simulink model "ame532Project1_onedrive"  (R2022a)
settings: Solver=ode4  StartTime=0.0  StopTime=120  FixedStep=0.01  RelTol=1e-3
model workspace (MAT data in the model file):
  theta = Simulink.Parameter
  theta.DataType = 'auto'
  theta.Complexity = 'real'
  theta.Dimensions = [0 0]
undefined symbols (not defined in the file): earthRadius
libraries: simulink_extras x11, matrix_library x6, aerolibfltsims x2, vrlib x1, aerolibtransform2 x1, aerolibutil x1
(part 1 of 2)
settings Model: Creator=enson  LastModifiedBy=enson

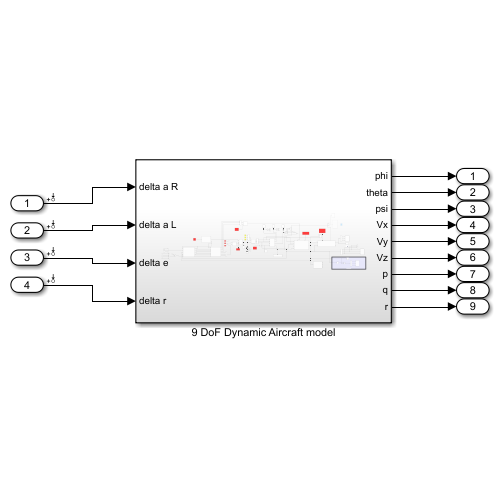
[thumbnail: Simulink's stored preview of the top-level diagram]
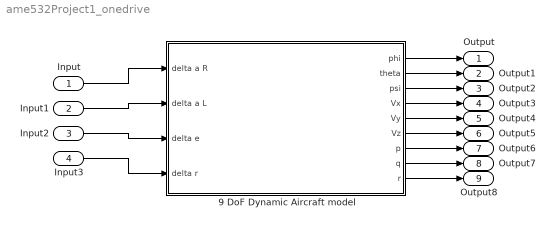
== system ame532Project1_onedrive ==
  Input : Inport
  Input1 : Inport  Port=2
  Input2 : Inport  Port=3
  Input3 : Inport  Port=4
  9 DoF Dynamic Aircraft model : Subsystem
  Output : Outport
  Output1 : Outport  Port=2
  Output2 : Outport  Port=3
  Output3 : Outport  Port=4
  Output4 : Outport  Port=5
  Output5 : Outport  Port=6
  Output6 : Outport  Port=7
  Output7 : Outport  Port=8
  Output8 : Outport  Port=9
  wires:
  Input/1 -> 9 DoF Dynamic Aircraft model/1(delta a R)
  Input1/1 -> 9 DoF Dynamic Aircraft model/2(delta a L)
  Input2/1 -> 9 DoF Dynamic Aircraft model/3(delta e)
  Input3/1 -> 9 DoF Dynamic Aircraft model/4(delta r)
  9 DoF Dynamic Aircraft model/1(phi) -> Output/1
  9 DoF Dynamic Aircraft model/2(theta) -> Output1/1
  9 DoF Dynamic Aircraft model/3(psi) -> Output2/1
  9 DoF Dynamic Aircraft model/4(Vx) -> Output3/1
  9 DoF Dynamic Aircraft model/5(Vy) -> Output4/1
  9 DoF Dynamic Aircraft model/6(Vz) -> Output5/1
  9 DoF Dynamic Aircraft model/7(p) -> Output6/1
  9 DoF Dynamic Aircraft model/8(q) -> Output7/1
  9 DoF Dynamic Aircraft model/9(r) -> Output8/1

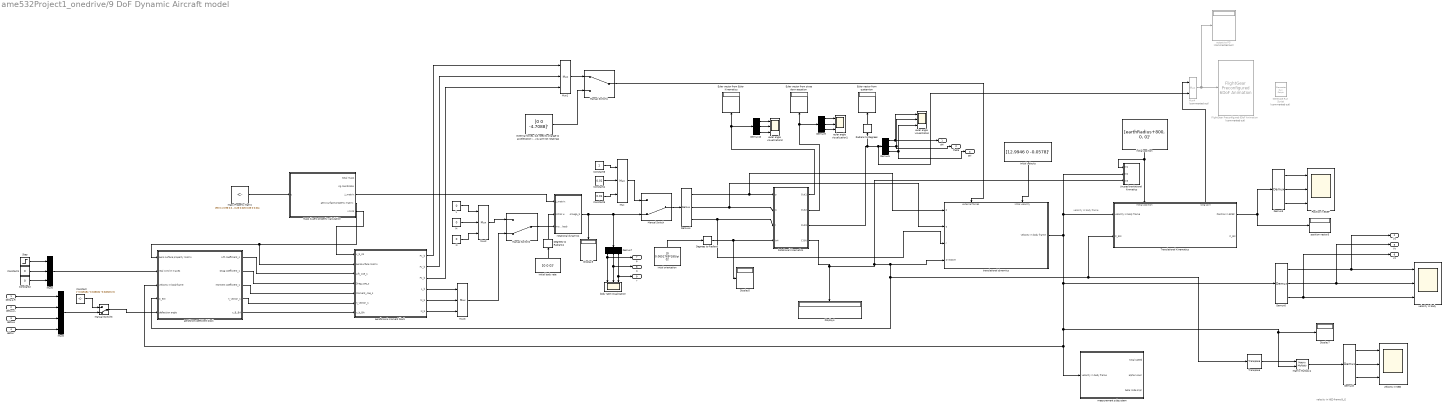
== system ame532Project1_onedrive/9 DoF Dynamic Aircraft model ==
  note: velocity in NED frame B_E
  note: velocity in body frame
  delta a R : Inport
  delta a L : Inport  Port=2
  delta e : Inport  Port=3
  delta r : Inport  Port=4
  Constant : Constant  Value=[-0.046184 -0.046184 -0.048101 0]
  Constant1 : Constant  Value=0
  Constant2 : Constant  Value=0
  Constant4 : Constant  Value=0.01
  Constant5 : Constant  Value=0.01
  Constant6 : Constant
  Degrees to Radians : simulink_extras/Transformations/Degrees to Radians
  Degrees to Radians1 : simulink_extras/Transformations/Degrees to Radians
  Demux{3..10} (8 alike) : Demux  Outputs=3
  Display{3..5,7} (4 alike) : Display
  Euler vector from Euler Kinematics : Display
  Euler vector from quaternion : Display
  Euler vector from strap down equation : Display
  FlightGear Preconfigured 6DoF Animation : aerolibfltsims/FlightGear Preconfigured 6DoF Animation  Commented=on  xFlightGearVersion=v2019.1  DestinationIpAddress=127.0.0.1  DestinationPort=5502  SampleTime=-1  packetVersion=24
  Generate Run Script : aerolibfltsims/Generate Run Script  Commented=on  Architecture=Win64  dataFlow=Send  GeometryModelName=c172p  AirportId=KSFO  RunwayId=10L  InitialAltitude=7224  InitialHeading=113  OffsetDistance=4.72  OffsetAzimuth=0  InstallScenery=off  DisableShaders=off  OriginAddress=127.0.0.1  DestinationPort=5502  OriginPort=5505  LocalAddress=127.0.0.1  OutputFileName=runfg.bat  FlightGearBaseDirectory=C:\Program Files\FlightGear 2020.3
  Initial body rate : Constant  Value=[0 0 0]'
  L : Constant  Value=0
  M : Constant  Value=0
  Manual Switch : ManualSwitch  CurrentSetting=0
  Manual Switch1 : ManualSwitch
  Manual Switch2 : ManualSwitch  CurrentSetting=0
  Manual Switch3 : ManualSwitch  CurrentSetting=0
  Mass Property Matrix : Constant  Value=|
      | [90 0.1 0.96 0.01 -0.23 0.44 0; 
      |  90 0.1 0.96 0.01 -0.23 -0.44 0; 
      |  13 0.075 0.35 0.002 -0.76 0 -0.16;
      |  0 0.08 0.002 0.18 -0.76 0 -0.09; 
      |  72 0.065 0.035 0.015 -0.05 0 0.03;
      |  106 0.87 0.07 0.07 -0.4 0 0;
      |  27 0.05 0.03 0.005 -0.05 0 0.02; 
      |  10 0.04 0.02 0.005 -0.1 0 0.02;
      |  20 0.05 0.01 0.01 -0.014 0 0; 
      |  40 0.03 0.02 0.02 0.02 0 0.01; 
      |  12 0 0.26 0.025 0.05 0 0.01];
  Matrix Multiply4 : Product  Multiplication=Matrix(*)
  Mux{,1..3,5} (5 alike) : Mux  Inputs=3
  Mux4 : Mux  Commented=on  Inputs=2
  Mux6 : Mux
  N : Constant  Value=0
  Position in ECEF : Scope  NumInputPorts=3
  Radians to Degrees : simulink_extras/Transformations/Radians to Degrees
  Rotational Kinematics : Subsystem
  Step : Step  Time=30  After=0  SampleTime=0
  Translational Kinematics : Subsystem
      settings: PortSchema="{\"entries\":[{\"content\":{\"sides\":[{\"content\":{\"connectorIds\":[\"In1\",\"In2\"]},\"type\":\"ConnectorPlacement.EquallySpacedRectSide\",\"uuid\":\"6a5083c9-3149-4656-b001-28ffe3d04409\"},{\"content\":{\"connectorIds\":[\"Out1\",\"Out2\"],\"side\":\"RIGHT\"},\"type\":\"ConnectorPlacement.EquallySpacedRectSide\",\"uuid\":\"fa51dba7-7f70-4cf9-abef-b6efe75fc937\"},{\"content\":{\"connectorIds\":[\"In3\",\"Out3\"],\"side\":\"TOP\"},\"type\":\"ConnectorPlacement.EquallySpacedRectSide\",\"uuid\":\"76f1511e-a5f6-41ee-949f-b44acacf362b\"}]},\"type\":\"ConnectorPlacement.EquallySpacedConnector\",\"uuid\":\"9a334045-2485-41ee-8c4a-be73d098fd92\"}],\"packageUris\":[\"http://schema.mathworks.com/mf0/Connector/R2020b\"],\"version\":\"1.0\"}"
  Transpose : matrix_library/Transpose
      settings: SourceProductBaseCode=SL
  Unused tranlational kinmatics : Subsystem
  aeroforce & moment block : Subsystem
  aeroforce coefficient block : Subsystem
  body rate visualization : Scope  NumInputPorts=3
  euler angle visualization : Scope  NumInputPorts=3
  euler angle visualization1 : Scope  NumInputPorts=3
  euler angle visualization2 : Scope  NumInputPorts=3
  "external forces, but need to change to acceleration in body these terms should also be corrected with DCM unless you are not rotating1" : Constant  Value=[0 0 -4.7088]'
  initial posiiton : Constant  Value=[earthRadius+800, 0, 0]'  VectorParams1D=off
  initial velocity : Constant  Value=[12.9946 0 -0.0578]'
  intial orientation : Constant  Value=[0 0.0651769*180/pi 0]'  VectorParams1D=off
  mass & aero property calculation : Subsystem
  measurement subsystem : Subsystem
  output to FG : Display  Commented=on
  position vector3 : Display
  rotational dynamics : Subsystem
  translational dynamics : Subsystem
      settings: PortSchema="{\"entries\":[{\"content\":{\"sides\":[{\"content\":{\"connectorIds\":[\"In1\",\"In2\",\"In3\",\"In4\"]},\"type\":\"ConnectorPlacement.EquallySpacedRectSide\",\"uuid\":\"eb52c09d-c71f-42a1-8e21-86a86e354291\"},{\"content\":{\"connectorIds\":[\"Out1\"],\"side\":\"RIGHT\"},\"type\":\"ConnectorPlacement.EquallySpacedRectSide\",\"uuid\":\"c050fdd0-50ab-42c8-8490-bbe72862ad59\"},{\"content\":{\"connectorIds\":[\"In5\",\"In6\"],\"side\":\"TOP\"},\"type\":\"ConnectorPlacement.EquallySpacedRectSide\",\"uuid\":\"d308cee2-bf9d-4ab9-b003-c94f4b2955f2\"},{\"content\":{\"connectorIds\":[],\"side\":\"BOTTOM\"},\"type\":\"ConnectorPlacement.EquallySpacedRectSide\",\"uuid\":\"cf51bcec-71dd-45f1-b1ae-be572a1ab1ac\"}]},\"type\":\"ConnectorPlacement.EquallySpacedConnector\",\"uuid\":\"72e461db-b4a1-4e87-8f9d-278a55fe116d\"}],\"packageUris\":[\"http://schema.mathworks.com/mf0/Connector/R2020b\"],\"version\":\"1.0\"}"
  velocity in NED : Scope  NumInputPorts=3
  velocity in body : Scope  NumInputPorts=3
  phi : Outport
  theta : Outport  Port=2
  psi : Outport  Port=3
  Vx : Outport  Port=4
  Vy : Outport  Port=5
  Vz : Outport  Port=6
  p : Outport  Port=7
  q : Outport  Port=8
  r : Outport  Port=9
  wires:
  Radians to Degrees/1 -> Euler vector from quaternion/1
  Demux6/2 -> Vy/1, velocity in body/2
  Matrix Multiply4/1 -> Demux8/1
  Constant2/1 -> Mux5/3
  "external forces, but need to change to acceleration in body these terms should also be corrected with DCM unless you are not rotating1"/1 -> Manual Switch1/2
  mass & aero property calculation/5(x b sb) -> aeroforce & moment block/1(x_b_sb)
  Demux3/2 -> Position in ECEF/2
  Demux8/2 -> velocity in NED/2
  Demux4/2 -> Rotational Kinematics/2(q), translational dynamics/2(q)
  Demux5/1 -> euler angle visualization/1, phi/1
  Demux10/1 -> euler angle visualization2/1
  Constant1/1 -> Mux5/2
  intial orientation/1 -> Degrees to Radians/1
  Demux8/3 -> velocity in NED/3
  Constant6/1 -> Mux/1
  Step/1 -> Mux5/1
  Rotational Kinematics/3(Out3) -> Mux4/2, Demux5/1, Radians to Degrees/1
  Manual Switch1/1 -> translational dynamics/5(external forces)
  Mux1/1 -> Manual Switch1/1
  initial posiiton/1 -> Unused tranlational kinmatics/1(In1), Translational Kinematics/3(initial position)
  Demux3/3 -> Position in ECEF/3
  Degrees to Radians/1 -> Display5/1, Rotational Kinematics/4(In4)
  Manual Switch/1 -> Demux4/1
  aeroforce & moment block/6(N_b) -> Mux3/3
  Demux4/1 -> translational dynamics/1(p), Rotational Kinematics/1(p)
  Degrees to Radians1/1 -> rotational dynamics/2(Initial w)
  Demux9/1 -> euler angle visualization1/1
  aeroforce & moment block/3(Fz_b) -> Mux1/3
  mass & aero property calculation/4(aero surface property matrix) -> aeroforce & moment block/2(aerosurface matrix), aeroforce coefficient block/1(aero surface property matrix)
  Demux3/1 -> Position in ECEF/1
  Translational Kinematics/1(Position in ECEF) -> position vector3/1, Demux3/1
  Demux4/3 -> translational dynamics/3(r), Rotational Kinematics/3(r)
  Manual Switch2/1 -> rotational dynamics/3(moment in body)
  Rotational Kinematics/1(Out1) -> Demux10/1, Euler vector from Euler Kinematics/1
  Demux10/3 -> euler angle visualization2/3
  aeroforce & moment block/5(M_b) -> Mux3/2
  Rotational Kinematics/2(Out2) -> Euler vector from strap down equation/1, Demux9/1
  Mux4/1 -> output to FG/1, FlightGear Preconfigured 6DoF Animation/1
  Translational Kinematics/3(long lat h) -> Mux4/1
  Demux10/2 -> euler angle visualization2/2
  Demux6/3 -> Vz/1, velocity in body/3
  Mux2/1 -> Manual Switch2/1
  aeroforce & moment block/2(Fy_b) -> Mux1/2
  mass & aero property calculation/3(J_matrix) -> rotational dynamics/1(J_matrix)
  Demux7/2 -> q/1, body rate visualization/2
  translational dynamics/1(velocity in body frame) -> measurement subsystem/1(velocity in body frame), aeroforce coefficient block/3(velocity in bodyframe), Matrix Multiply4/2, Display7/1, Demux6/1, Translational Kinematics/1(velocity in body frame), Unused tranlational kinmatics/2(In2)
  Rotational Kinematics/4(C BN) -> Display4/1, Unused tranlational kinmatics/3(In3), Transpose/1, Translational Kinematics/2(C_BN), aeroforce coefficient block/4(C_BN), translational dynamics/4(ZYXDCM)
  Mass Property Matrix/1 -> mass & aero property calculation/1(u)
  Demux5/3 -> psi/1, euler angle visualization/3
  Demux5/2 -> theta/1, euler angle visualization/2
  aeroforce coefficient block/2(Drag coefficient_s) -> aeroforce & moment block/4(Drag_coe_s)
  initial velocity/1 -> translational dynamics/6(intial velocity)
  Constant5/1 -> Mux/3
  M/1 -> Mux2/2
  aeroforce coefficient block/1(Lift coefficient_s) -> aeroforce & moment block/3(Lift_coe_s)
  Constant4/1 -> Mux/2
  rotational dynamics/1(omega_b) -> Manual Switch/2, Demux7/1, Display3/1
  Demux7/3 -> r/1, body rate visualization/3
  aeroforce & moment block/1(Fx_b) -> Mux1/1
  aeroforce & moment block/4(L_b) -> Mux3/1
  Mux5/1 -> aeroforce coefficient block/2(real wind in N axes)
  Demux8/1 -> velocity in NED/1
  Demux7/1 -> body rate visualization/1, p/1
  L/1 -> Mux2/1
  aeroforce coefficient block/3(Moment coefficient_s) -> aeroforce & moment block/5(Moment_coe_s)
  Demux9/2 -> euler angle visualization1/2
  Mux/1 -> Manual Switch/1
  Transpose/1 -> Matrix Multiply4/1
  Mux3/1 -> Manual Switch2/2
  Initial body rate/1 -> Degrees to Radians1/1
  Demux9/3 -> euler angle visualization1/3
  aeroforce coefficient block/4(n_vector_s) -> aeroforce & moment block/6(n_vector_s)
  aeroforce coefficient block/5(v_B_BA) -> aeroforce & moment block/7(v_b_BA)
  Demux6/1 -> Vx/1, velocity in body/1
  N/1 -> Mux2/3
  delta a R/1 -> Mux6/1
  delta a L/1 -> Mux6/2
  delta e/1 -> Mux6/3
  delta r/1 -> Mux6/4
  Manual Switch3/1 -> aeroforce coefficient block/5(deflection angle)
  Mux6/1 -> Manual Switch3/2
  Constant/1 -> Manual Switch3/1

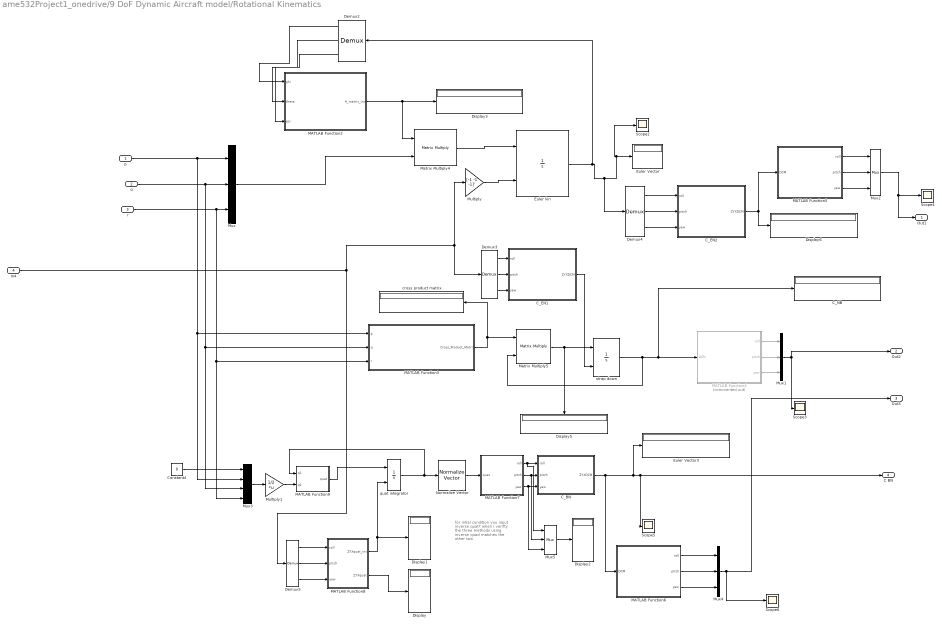
== system ame532Project1_onedrive/9 DoF Dynamic Aircraft model/Rotational Kinematics ==
  note: for intial condition you input inverse quat?
      | when I verifty the three methods using inverse quad matches the other two
  p : Inport
  q : Inport  Port=2
  r : Inport  Port=3
  In4 : Inport  Port=4
  C_BN : MATLAB Function  TreatAsAtomicUnit=on
  C_EN1 : MATLAB Function  TreatAsAtomicUnit=on
  C_EN2 : MATLAB Function  TreatAsAtomicUnit=on
  C_NB : Display
  Constant4 : Constant  Value=0
  Demux{2..5} (4 alike) : Demux  Outputs=3
  Display{,1..3,5..6} (6 alike) : Display
  Euler Vector : Display
  Euler Vector3 : Display
  Euler kin : Integrator  InitialConditionSource=external
  MATLAB Function2 : MATLAB Function  TreatAsAtomicUnit=on
  MATLAB Function3 : MATLAB Function  TreatAsAtomicUnit=on
  MATLAB Function4 : MATLAB Function  Commented=on  TreatAsAtomicUnit=on
  MATLAB Function5 : MATLAB Function  TreatAsAtomicUnit=on
  MATLAB Function6 : MATLAB Function  TreatAsAtomicUnit=on
  MATLAB Function7 : MATLAB Function  TreatAsAtomicUnit=on
  MATLAB Function8 : MATLAB Function  TreatAsAtomicUnit=on
  MATLAB Function9 : MATLAB Function  TreatAsAtomicUnit=on
  Matrix Multiply4 : Product  Multiplication=Matrix(*)
  Matrix Multiply5 : Product  Multiplication=Matrix(*)
  Multiply : Gain  Gain=[-1 -1 -1]'
  Multiply1 : Gain  Gain=1/2  Multiplication=Matrix(K*u)
  Mux{,1..2,4..5} (5 alike) : Mux  Inputs=3
  Mux3 : Mux
  Normalize Vector : vrlib/Utilities/Normalize Vector  maxzero=0
  Scope{2..6} (5 alike) : Scope
  cross product matrix : Display
  quat integrator : Integrator  InitialConditionSource=external  InitialCondition=[1 0 0 0]'
  strap down : Integrator  InitialConditionSource=external
  Out1 : Outport
  Out2 : Outport  Port=2
  Out3 : Outport  Port=3
  C BN : Outport  Port=4
  wires:
  Matrix Multiply4/1 -> Euler kin/1
  In4/1 -> Multiply/1, Demux3/1, Demux5/1
  MATLAB Function4/3(yaw) -> Mux1/3
  Euler kin/1 -> Scope2/1, Euler Vector/1, Demux4/1, Demux2/1
  MATLAB Function2/1(H_matrix_inv) -> Display3/1, Matrix Multiply4/1
  MATLAB Function6/2(pitch) -> Mux4/2
  r/1 -> Mux3/4, MATLAB Function3/3(r), Mux/3
  Matrix Multiply5/1 -> Display5/1, strap down/1
  Mux/1 -> Matrix Multiply4/2
  q/1 -> Mux3/3, MATLAB Function3/2(q), Mux/2
  C_BN/1(ZYXDCM) -> MATLAB Function6/1(DCM), C BN/1, Scope5/1, Euler Vector3/1
  C_EN1/1(ZYXDCM) -> strap down/2
  MATLAB Function5/2(pitch) -> Mux2/2
  Mux1/1 -> Out2/1, Scope3/1
  MATLAB Function4/1(roll) -> Mux1/1
  Demux2/2 -> MATLAB Function2/2(theta)
  Demux4/3 -> C_EN2/3(yaw)
  MATLAB Function4/2(pitch) -> Mux1/2
  Demux2/3 -> MATLAB Function2/3(psi)
  Demux2/1 -> MATLAB Function2/1(phi)
  Demux5/1 -> MATLAB Function8/1(roll)
  Demux3/1 -> C_EN1/1(roll)
  Demux5/2 -> MATLAB Function8/2(pitch)
  Demux4/1 -> C_EN2/1(roll)
  Demux3/3 -> C_EN1/3(yaw)
  Multiply/1 -> Euler kin/2
  C_EN2/1(ZYXDCM) -> Display6/1, MATLAB Function5/1(DCM)
  Normalize Vector/1 -> MATLAB Function7/1(quat)
  MATLAB Function9/1(quat) -> quat integrator/1
  strap down/1 -> Matrix Multiply5/2, MATLAB Function4/1(DCM), C_NB/1
  p/1 -> Mux3/2, MATLAB Function3/1(p), Mux/1
  quat integrator/1 -> Normalize Vector/1, MATLAB Function9/1(q1)
  MATLAB Function7/3(yaw) -> Mux5/3, C_BN/3(yaw)
  Mux2/1 -> Out1/1, Scope4/1
  MATLAB Function5/3(yaw) -> Mux2/3
  Constant4/1 -> Mux3/1
  Mux3/1 -> Multiply1/1
  Mux4/1 -> Out3/1, Scope6/1
  MATLAB Function7/1(roll) -> Mux5/1, C_BN/1(roll)
  MATLAB Function5/1(roll) -> Mux2/1
  Demux5/3 -> MATLAB Function8/3(yaw)
  MATLAB Function6/1(roll) -> Mux4/1
  MATLAB Function6/3(yaw) -> Mux4/3
  Multiply1/1 -> MATLAB Function9/2(q2)
  MATLAB Function3/1(Cross_Product_Matrix) -> Matrix Multiply5/1, cross product matrix/1
  Demux4/2 -> C_EN2/2(pitch)
  Demux3/2 -> C_EN1/2(pitch)
  MATLAB Function7/2(pitch) -> Mux5/2, C_BN/2(pitch)
  MATLAB Function8/1(ZYXquat_inv) -> quat integrator/2, Display1/1
  MATLAB Function8/2(ZYXquat) -> Display/1
  Mux5/1 -> Display2/1

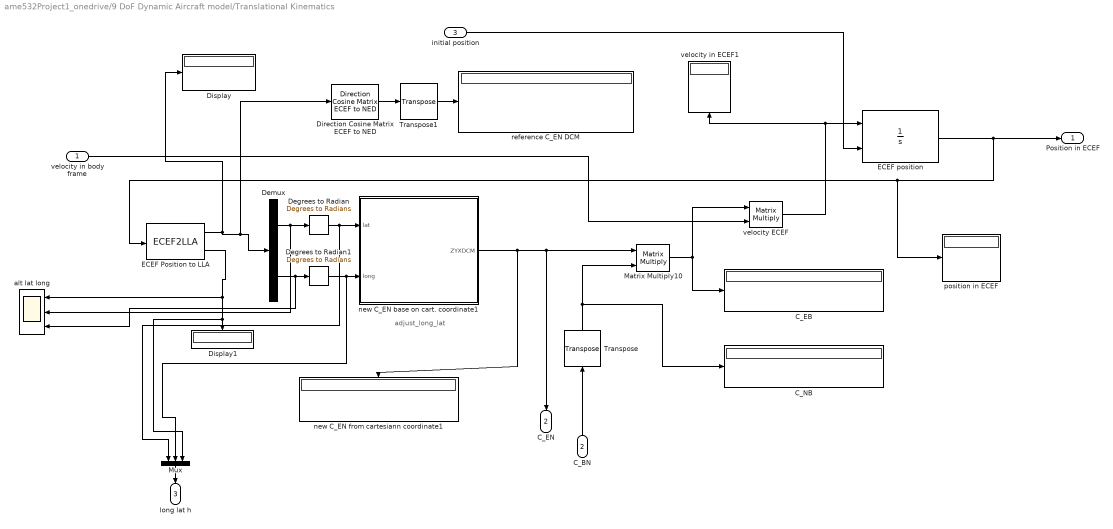
== system ame532Project1_onedrive/9 DoF Dynamic Aircraft model/Translational Kinematics ==
  note: adjust_long_lat
  velocity in body frame : Inport
  C_BN : Inport  Port=2
  initial position : Inport  Port=3
  C_EB : Display
  C_NB : Display
  Degrees to Radian : simulink_extras/Transformations/Degrees to Radians
  Degrees to Radian1 : simulink_extras/Transformations/Degrees to Radians
  Demux : Demux  Outputs=2
  Direction Cosine Matrix ECEF to NED : aerolibtransform2/Direction Cosine Matrix ECEF to NED
      settings: SourceProductBaseCode=AE
  Display : Display
  Display1 : Display
  ECEF Position to LLA : ECEF2LLA  ptype=Custom  R=earthRadius
  ECEF position : Integrator  InitialConditionSource=external  InitialCondition=[6378100,0,0]'
  Matrix Multiply10 : Product  Multiplication=Matrix(*)
  Mux : Mux  Inputs=3
  Transpose : matrix_library/Transpose
      settings: SourceProductBaseCode=SL
  Transpose1 : matrix_library/Transpose
      settings: SourceProductBaseCode=SL
  alt lat long : Scope  NumInputPorts=3
  new C_EN base on cart. coordinate1 : MATLAB Function  TreatAsAtomicUnit=on
  new C_EN from cartesiann coordinate1 : Display
  position in ECEF : Display
  reference C_EN DCM : Display
  velocity ECEF : Product  Multiplication=Matrix(*)
  velocity in ECEF1 : Display
  Position in ECEF : Outport
  C_EN : Outport  Port=2
  long lat h : Outport  Port=3
  wires:
  ECEF position/1 -> Position in ECEF/1, ECEF Position to LLA/1, position in ECEF/1
  initial position/1 -> ECEF position/2
  new C_EN base on cart. coordinate1/1(ZYXDCM) -> new C_EN from cartesiann coordinate1/1, C_EN/1, Matrix Multiply10/1
  Matrix Multiply10/1 -> C_EB/1, velocity ECEF/1
  velocity ECEF/1 -> ECEF position/1, velocity in ECEF1/1
  velocity in body frame/1 -> velocity ECEF/2
  C_BN/1 -> Transpose/1
  ECEF Position to LLA/1 -> Direction Cosine Matrix ECEF to NED/1, Demux/1, Display/1
  ECEF Position to LLA/2 -> alt lat long/1, Mux/3, Display1/1
  Demux/1 -> Degrees to Radian/1, alt lat long/2
  Demux/2 -> alt lat long/3, Degrees to Radian1/1
  Degrees to Radian/1 -> Mux/1, new C_EN base on cart. coordinate1/1(lat)
  Degrees to Radian1/1 -> Mux/2, new C_EN base on cart. coordinate1/2(long)
  Transpose/1 -> C_NB/1, Matrix Multiply10/2
  Direction Cosine Matrix ECEF to NED/1 -> Transpose1/1
  Transpose1/1 -> reference C_EN DCM/1
  Mux/1 -> long lat h/1

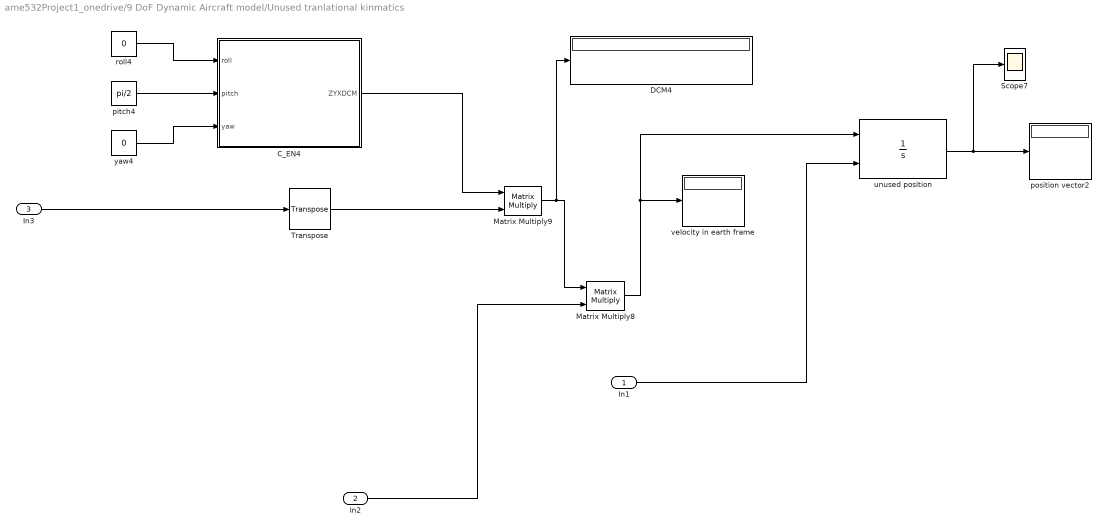
== system ame532Project1_onedrive/9 DoF Dynamic Aircraft model/Unused tranlational kinmatics ==
  In1 : Inport
  In2 : Inport  Port=2
  In3 : Inport  Port=3
  C_EN4 : MATLAB Function  TreatAsAtomicUnit=on
  DCM4 : Display
  Matrix Multiply8 : Product  Multiplication=Matrix(*)
  Matrix Multiply9 : Product  Multiplication=Matrix(*)
  Scope7 : Scope
  Transpose : matrix_library/Transpose
      settings: SourceProductBaseCode=SL
  pitch4 : Constant  Value=pi/2
  position vector2 : Display
  roll4 : Constant  Value=0
  unused position : Integrator  InitialConditionSource=external  InitialCondition=[6378100,0,0]'
  velocity in earth frame : Display
  yaw4 : Constant  Value=0
  wires:
  Matrix Multiply9/1 -> DCM4/1, Matrix Multiply8/1
  unused position/1 -> Scope7/1, position vector2/1
  C_EN4/1(ZYXDCM) -> Matrix Multiply9/1
  Matrix Multiply8/1 -> velocity in earth frame/1, unused position/1
  yaw4/1 -> C_EN4/3(yaw)
  pitch4/1 -> C_EN4/2(pitch)
  Transpose/1 -> Matrix Multiply9/2
  roll4/1 -> C_EN4/1(roll)
  In2/1 -> Matrix Multiply8/2
  In1/1 -> unused position/2
  In3/1 -> Transpose/1

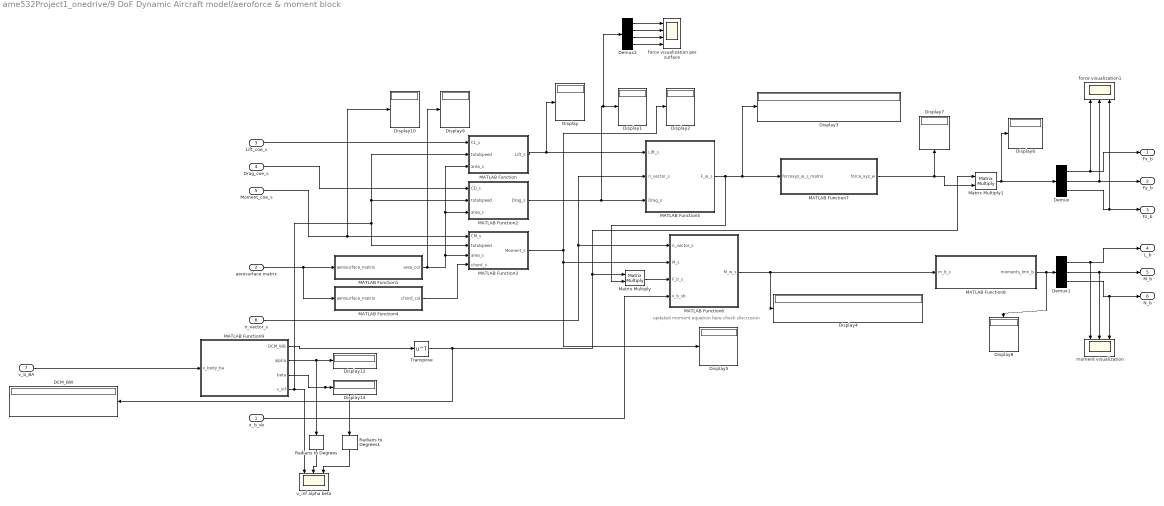
== system ame532Project1_onedrive/9 DoF Dynamic Aircraft model/aeroforce & moment block ==
  note: updated moment equation here check disccusion
  x_b_sb : Inport
  aerosurface matrix : Inport  Port=2
  Lift_coe_s : Inport  Port=3
  Drag_coe_s : Inport  Port=4
  Moment_coe_s : Inport  Port=5
  n_vector_s : Inport  Port=6
  v_b_BA : Inport  Port=7
  DCM_BW : Display
  Demux : Demux  Outputs=3
  Demux1 : Demux  Outputs=3
  Demux2 : Demux
  Display{,1..10,12,14} (13 alike) : Display
  MATLAB Function : MATLAB Function  TreatAsAtomicUnit=on
  MATLAB Function1 : MATLAB Function  TreatAsAtomicUnit=on
  MATLAB Function2 : MATLAB Function  TreatAsAtomicUnit=on
  MATLAB Function3 : MATLAB Function  TreatAsAtomicUnit=on
  MATLAB Function4 : MATLAB Function  TreatAsAtomicUnit=on
  MATLAB Function5 : MATLAB Function  TreatAsAtomicUnit=on
  MATLAB Function6 : MATLAB Function  TreatAsAtomicUnit=on
  MATLAB Function7 : MATLAB Function  TreatAsAtomicUnit=on
  MATLAB Function8 : MATLAB Function  TreatAsAtomicUnit=on
  MATLAB Function9 : MATLAB Function  TreatAsAtomicUnit=on
  Matrix Multiply : Product  Multiplication=Matrix(*)
  Matrix Multiply1 : Product  Multiplication=Matrix(*)
  Radians to Degrees : simulink_extras/Transformations/Radians to Degrees
  Radians to Degrees1 : simulink_extras/Transformations/Radians to Degrees
  Transpose : Math  Operator=transpose
  force visualization per surface : Scope  NumInputPorts=4
  force visualization1 : Scope  NumInputPorts=3
  moment visualization : Scope  NumInputPorts=3
  v_inf alpha beta : Scope  NumInputPorts=3
  Fx_b : Outport
  Fy_b : Outport  Port=2
  Fz_b : Outport  Port=3
  L_b : Outport  Port=4
  M_b : Outport  Port=5
  N_b : Outport  Port=6
  wires:
  Lift_coe_s/1 -> MATLAB Function/1(CL_s)
  MATLAB Function9/4(v_inf) -> v_inf alpha beta/1, MATLAB Function2/2(totalspeed), MATLAB Function/2(totalspeed), MATLAB Function3/2(totalspeed)
  aerosurface matrix/1 -> MATLAB Function4/1(aerosurface_matrix), MATLAB Function1/1(aerosurface_matrix)
  MATLAB Function1/1(area_col) -> Display9/1, MATLAB Function2/3(area_s), MATLAB Function/3(area_s), MATLAB Function3/3(area_s)
  Drag_coe_s/1 -> MATLAB Function2/1(CD_s)
  Moment_coe_s/1 -> Display10/1, MATLAB Function3/1(CM_s)
  MATLAB Function4/1(chord_col) -> MATLAB Function3/4(chord_s)
  n_vector_s/1 -> MATLAB Function5/2(n_vector_s), MATLAB Function6/1(n_vector_s)
  MATLAB Function/1(Lift_s) -> Display/1, MATLAB Function5/1(Lift_s)
  MATLAB Function2/1(Drag_s) -> MATLAB Function5/3(Drag_s), Demux2/1, Display1/1
  MATLAB Function3/1(Moment_s) -> Display5/1, MATLAB Function6/2(M_s), Display2/1
  MATLAB Function6/1(M_w_s) -> Display4/1, MATLAB Function8/1(m_b_s)
  Matrix Multiply/1 -> MATLAB Function6/3(F_b_s)
  x_b_sb/1 -> MATLAB Function6/4(x_b_sb)
  MATLAB Function5/1(F_w_s) -> Matrix Multiply/2, Display3/1, MATLAB Function7/1(forcexyz_w_s_matrix)
  MATLAB Function7/1(force_xyz_w) -> Matrix Multiply1/2, Display7/1
  MATLAB Function8/1(moments_lmn_b) -> Demux1/1, Display8/1
  Matrix Multiply1/1 -> Demux/1, Display6/1
  MATLAB Function9/1(DCM_WB) -> Transpose/1
  v_b_BA/1 -> MATLAB Function9/1(v_body_ba)
  MATLAB Function9/2(alpha) -> Radians to Degrees/1, Display12/1
  MATLAB Function9/3(beta) -> Display14/1, Radians to Degrees1/1
  Demux1/1 -> L_b/1, moment visualization/1
  Demux1/2 -> M_b/1, moment visualization/2
  Demux1/3 -> moment visualization/3, N_b/1
  Demux/1 -> Fx_b/1, force visualization1/1
  Demux/2 -> Fy_b/1, force visualization1/2
  Demux/3 -> Fz_b/1, force visualization1/3
  Transpose/1 -> Matrix Multiply1/1, Matrix Multiply/1, DCM_BW/1
  Radians to Degrees/1 -> v_inf alpha beta/2
  Radians to Degrees1/1 -> v_inf alpha beta/3
  Demux2/4 -> force visualization per surface/4
  Demux2/3 -> force visualization per surface/3
  Demux2/2 -> force visualization per surface/2
  Demux2/1 -> force visualization per surface/1

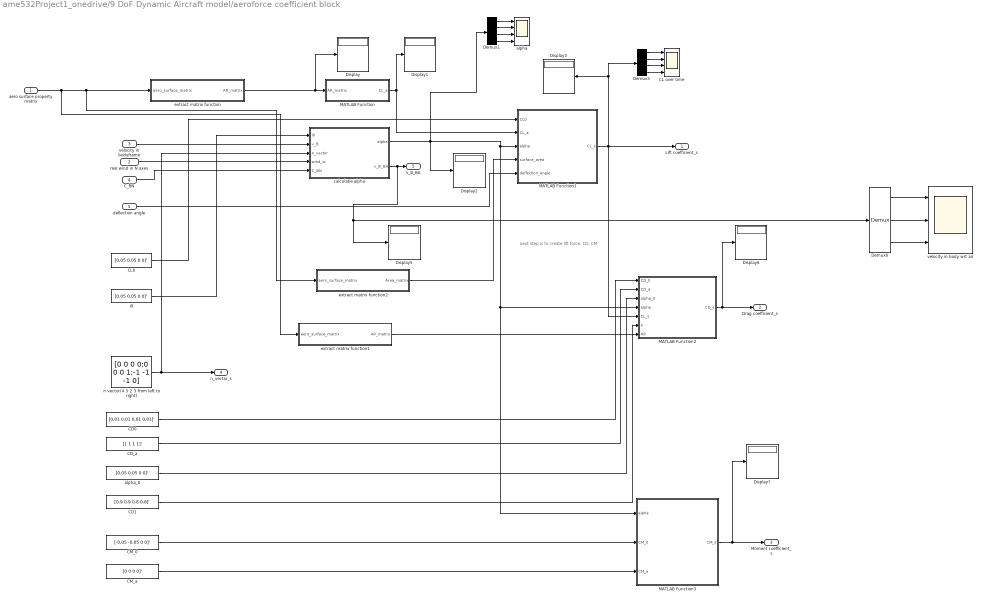
== system ame532Project1_onedrive/9 DoF Dynamic Aircraft model/aeroforce coefficient block ==
  note: next step is to create lift force, CD, CM
  aero surface property matrix : Inport
  real wind in N axes : Inport  Port=2
  velocity in bodyframe : Inport  Port=3
  C_BN : Inport  Port=4
  deflection angle : Inport  Port=5
  CD0 : Constant  Value=[0.01 0.01 0.01 0.01]'
  CD1 : Constant  Value=[0.9 0.9 0.8 0.8]'
  CD_a : Constant  Value=[1 1 1 1]'
  CL over time : Scope  NumInputPorts=4
  CL0 : Constant  Value=[0.05 0.05 0 0]'
  CM_0 : Constant  Value=[-0.05 -0.05 0 0]'
  CM_a : Constant  Value=[0 0 0 0]'
  Demux1 : Demux
  Demux5 : Demux
  Demux6 : Demux  Outputs=3
  Display{,1..3,5..7} (7 alike) : Display
  MATLAB Function : MATLAB Function  TreatAsAtomicUnit=on
  MATLAB Function1 : MATLAB Function  TreatAsAtomicUnit=on
  MATLAB Function2 : MATLAB Function  TreatAsAtomicUnit=on
  MATLAB Function3 : MATLAB Function  TreatAsAtomicUnit=on
  alpha : Scope  NumInputPorts=4
  alpha_0 : Constant  Value=[0.05 0.05 0 0]'
  calculatie alpha : MATLAB Function  TreatAsAtomicUnit=on
  extract matrix function : MATLAB Function  TreatAsAtomicUnit=on
  extract matrix function1 : MATLAB Function  TreatAsAtomicUnit=on
  extract matrix function2 : MATLAB Function  TreatAsAtomicUnit=on
  i0 : Constant  Value=[0.05 0.05 0 0]'
  n vector(4 5 2 3 from left to right) : Constant  Value=[0 0 0 0;0 0 0 1;-1 -1 -1 0]
  velocity in body wrt air : Scope  NumInputPorts=3
  Lift coefficient_s : Outport
  Drag coefficient_s : Outport  Port=2
  Moment coefficient_s : Outport  Port=3
  n_vector_s : Outport  Port=4
  v_B_BA : Outport  Port=5
  wires:
  aero surface property matrix/1 -> extract matrix function1/1(aero_surface_matrix), extract matrix function/1(aero_surface_matrix), extract matrix function2/1(aero_surface_matrix)
  extract matrix function/1(AR_matrix) -> Display/1, MATLAB Function/1(AR_matrix)
  MATLAB Function/1(CL_a) -> MATLAB Function1/2(CL_a), Display1/1
  n vector(4 5 2 3 from left to right)/1 -> n_vector_s/1, calculatie alpha/3(n_vector)
  velocity in bodyframe/1 -> calculatie alpha/2(v_B)
  i0/1 -> calculatie alpha/1(i0)
  CL0/1 -> MATLAB Function1/1(CL0)
  Demux5/2 -> CL over time/2
  Demux5/1 -> CL over time/1
  Demux5/3 -> CL over time/3
  MATLAB Function1/1(CL_s) -> Demux5/1, Display3/1, Lift coefficient_s/1, MATLAB Function2/5(CL_s)
  Demux5/4 -> CL over time/4
  real wind in N axes/1 -> calculatie alpha/4(wind_w)
  extract matrix function1/1(AR_matrix) -> MATLAB Function2/7(AR)
  CD1/1 -> MATLAB Function2/6(e)
  alpha_0/1 -> MATLAB Function2/3(alpha_0)
  CD0/1 -> MATLAB Function2/1(CD_0)
  CD_a/1 -> MATLAB Function2/2(CD_a)
  MATLAB Function2/1(CD_s) -> Drag coefficient_s/1, Display6/1
  CM_0/1 -> MATLAB Function3/2(CM_0)
  CM_a/1 -> MATLAB Function3/3(CM_a)
  MATLAB Function3/1(CM_s) -> Moment coefficient_s/1, Display7/1
  C_BN/1 -> calculatie alpha/5(C_BN)
  calculatie alpha/2(v_B_BA) -> Demux6/1, Display5/1, v_B_BA/1
  Demux6/3 -> velocity in body wrt air/3
  Demux6/2 -> velocity in body wrt air/2
  Demux6/1 -> velocity in body wrt air/1
  Demux1/1 -> alpha/1
  Demux1/2 -> alpha/2
  Demux1/3 -> alpha/3
  Demux1/4 -> alpha/4
  calculatie alpha/1(alpha) -> MATLAB Function3/1(alpha), MATLAB Function2/4(alpha), MATLAB Function1/3(alpha), Display2/1, Demux1/1
  extract matrix function2/1(Area_matrix) -> MATLAB Function1/4(surface_area)
  deflection angle/1 -> MATLAB Function1/5(deflection_angle)

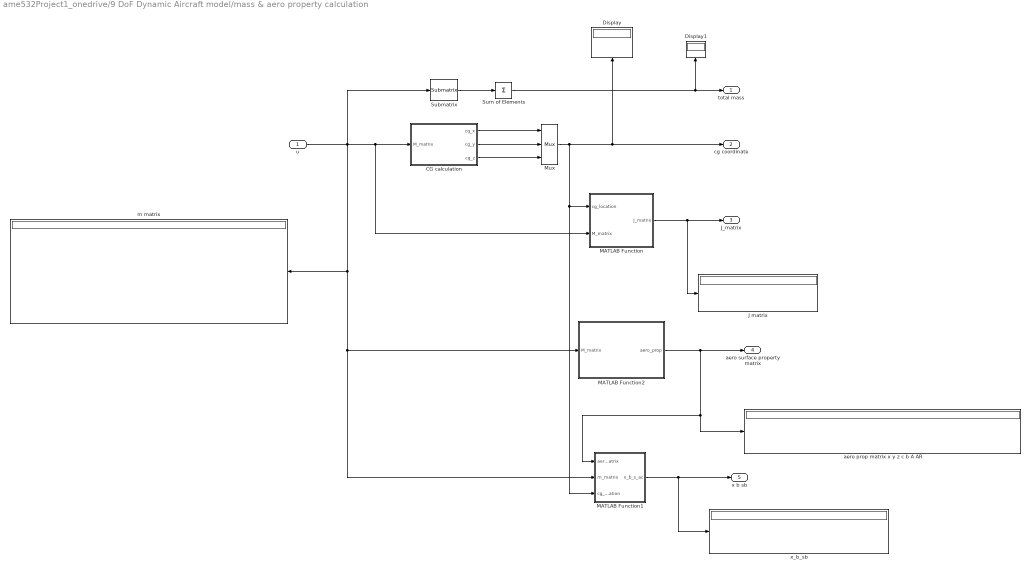
== system ame532Project1_onedrive/9 DoF Dynamic Aircraft model/mass & aero property calculation ==
  u : Inport
  CG calculation : MATLAB Function  TreatAsAtomicUnit=on
  Display : Display
  Display1 : Display
  J matrix : Display
  MATLAB Function : MATLAB Function  TreatAsAtomicUnit=on
  MATLAB Function1 : MATLAB Function  TreatAsAtomicUnit=on
  MATLAB Function2 : MATLAB Function  TreatAsAtomicUnit=on
  Mux : Mux  Inputs=3
  Submatrix : matrix_library/Submatrix  RowSpan=All rows  RowStartMode=First  RowStartIndex=1  RowEndMode=Last  RowEndIndex=1  ColSpan=One column  ColStartMode=First  ColStartIndex=1  ColEndMode=Last  ColEndIndex=1
      settings: SourceProductBaseCode=SL
  Sum of Elements : Sum  Inputs=+
  aero prop matrix x y z c b A AR : Display
  m matrix : Display
  x_b_sb : Display
  total mass : Outport
  cg coordinate : Outport  Port=2
  J_matrix : Outport  Port=3
  aero surface property matrix : Outport  Port=4
  x b sb : Outport  Port=5
  wires:
  CG calculation/1(cg_x) -> Mux/1
  u/1 -> MATLAB Function1/2(m_matrix), MATLAB Function2/1(M_matrix), m matrix/1, Submatrix/1, MATLAB Function/2(M_matrix), CG calculation/1(M_matrix)
  CG calculation/2(cg_y) -> Mux/2
  CG calculation/3(cg_z) -> Mux/3
  Mux/1 -> MATLAB Function1/3(cg_location), MATLAB Function/1(cg_location), cg coordinate/1, Display/1
  Submatrix/1 -> Sum of Elements/1
  Sum of Elements/1 -> total mass/1, Display1/1
  MATLAB Function/1(J_matrix) -> J_matrix/1, J matrix/1
  MATLAB Function2/1(aero_prop) -> MATLAB Function1/1(aero_prop_matrix), aero prop matrix x y z c b A AR/1, aero surface property matrix/1
  MATLAB Function1/1(x_b_s_ac) -> x b sb/1, x_b_sb/1

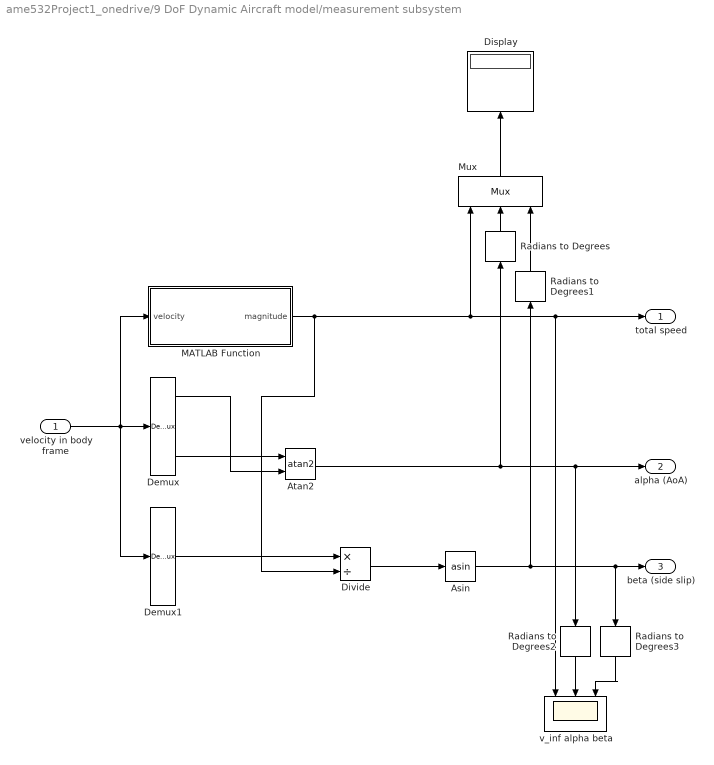
== system ame532Project1_onedrive/9 DoF Dynamic Aircraft model/measurement subsystem ==
  velocity in body frame : Inport
  Asin : Trigonometry  Operator=asin
  Atan2 : Trigonometry  Operator=atan2
  Demux : Demux  Outputs=3
  Demux1 : Demux  Outputs=3
  Display : Display
  Divide : Product  Inputs=*/  RndMeth=Zero  SaturateOnIntegerOverflow=on
  MATLAB Function : MATLAB Function  TreatAsAtomicUnit=on
  Mux : Mux  Inputs=3
  Radians to Degrees{,1..3} (4 alike) : simulink_extras/Transformations/Radians to Degrees
  v_inf alpha beta : Scope  NumInputPorts=3
  total speed : Outport
  alpha (AoA) : Outport  Port=2
  beta (side slip) : Outport  Port=3
  wires:
  MATLAB Function/1(magnitude) -> Divide/2, Mux/1, total speed/1, v_inf alpha beta/1
  velocity in body frame/1 -> MATLAB Function/1(velocity), Demux1/1, Demux/1
  Demux/3 -> Atan2/1
  Demux/1 -> Atan2/2
  Atan2/1 -> alpha (AoA)/1, Radians to Degrees2/1, Radians to Degrees/1
  Demux1/2 -> Divide/1
  Divide/1 -> Asin/1
  Asin/1 -> beta (side slip)/1, Radians to Degrees3/1, Radians to Degrees1/1
  Mux/1 -> Display/1
  Radians to Degrees/1 -> Mux/2
  Radians to Degrees1/1 -> Mux/3
  Radians to Degrees2/1 -> v_inf alpha beta/2
  Radians to Degrees3/1 -> v_inf alpha beta/3

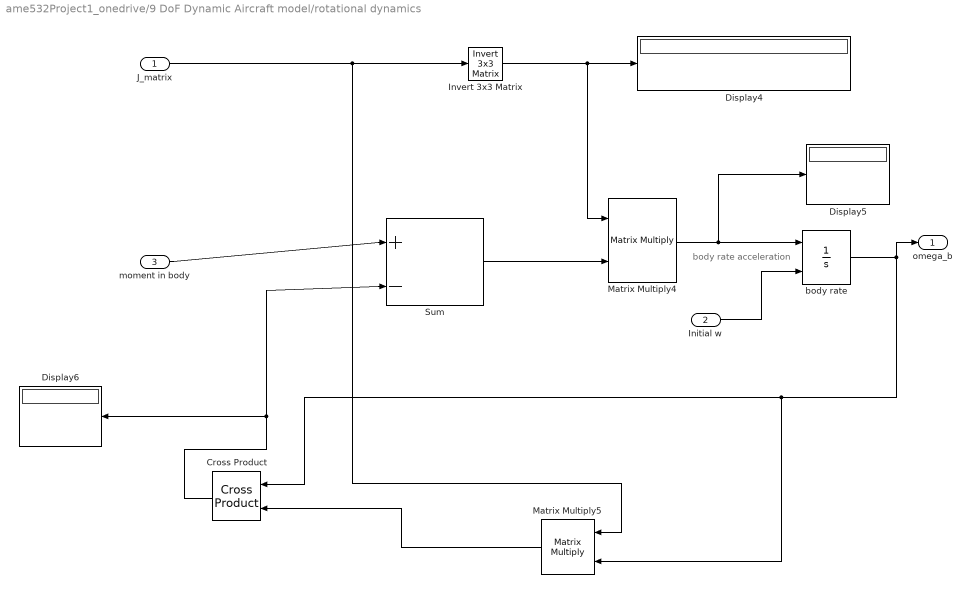
== system ame532Project1_onedrive/9 DoF Dynamic Aircraft model/rotational dynamics ==
  note: body rate acceleration
  J_matrix : Inport
  Initial w : Inport  Port=2
  moment in body : Inport  Port=3
  Cross Product : matrix_library/Cross Product
      settings: SourceProductBaseCode=SL
  Display4 : Display
  Display5 : Display
  Display6 : Display
  Invert 3x3 Matrix : aerolibutil/Invert  3x3 Matrix
  Matrix Multiply4 : Product  Multiplication=Matrix(*)
  Matrix Multiply5 : Product  Multiplication=Matrix(*)
  Sum : Sum  Inputs=|+-
  body rate : Integrator  InitialConditionSource=external  InitialCondition=[0 0 0]'
  omega_b : Outport
  wires:
  Cross Product/1 -> Sum/2, Display6/1
  Sum/1 -> Matrix Multiply4/2
  J_matrix/1 -> Matrix Multiply5/1, Invert 3x3 Matrix/1
  body rate/1 -> omega_b/1, Matrix Multiply5/2, Cross Product/1
  Matrix Multiply4/1 -> Display5/1, body rate/1
  Invert 3x3 Matrix/1 -> Matrix Multiply4/1, Display4/1
  Matrix Multiply5/1 -> Cross Product/2
  Initial w/1 -> body rate/2
  moment in body/1 -> Sum/1

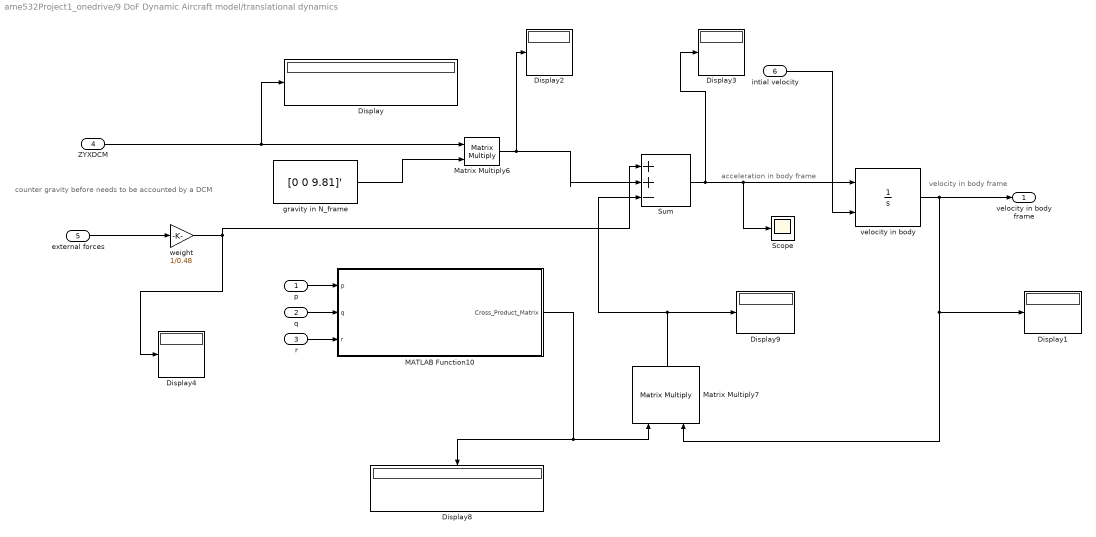
== system ame532Project1_onedrive/9 DoF Dynamic Aircraft model/translational dynamics ==
  note: counter gravity before needs to be accounted by a DCM
  note: velocity in body frame
  note: acceleration in body frame
  p : Inport
  q : Inport  Port=2
  r : Inport  Port=3
  ZYXDCM : Inport  Port=4
  external forces : Inport  Port=5
  intial velocity : Inport  Port=6
  Display{,1..4,8..9} (7 alike) : Display
  MATLAB Function10 : MATLAB Function  TreatAsAtomicUnit=on
  Matrix Multiply6 : Product  Multiplication=Matrix(*)
  Matrix Multiply7 : Product  Multiplication=Matrix(*)
  Scope : Scope
  Sum : Sum  Inputs=|++-
  gravity in N_frame : Constant  Value=[0 0 9.81]'
  "velocity in body " : Integrator  InitialConditionSource=external
  weight : Gain  Gain=1/0.48
  velocity in body frame : Outport
  wires:
  MATLAB Function10/1(Cross_Product_Matrix) -> Matrix Multiply7/1, Display8/1
  "velocity in body "/1 -> velocity in body frame/1, Display1/1, Matrix Multiply7/2
  Sum/1 -> Display3/1, Scope/1, "velocity in body "/1
  Matrix Multiply6/1 -> Sum/2, Display2/1
  Matrix Multiply7/1 -> Sum/3, Display9/1
  ZYXDCM/1 -> Display/1, Matrix Multiply6/1
  q/1 -> MATLAB Function10/2(q)
  p/1 -> MATLAB Function10/1(p)
  r/1 -> MATLAB Function10/3(r)
  intial velocity/1 -> "velocity in body "/2
  gravity in N_frame/1 -> Matrix Multiply6/2
  external forces/1 -> weight/1
  weight/1 -> Sum/1, Display4/1

== matlab function ame532Project1_onedrive/9 DoF Dynamic Aircraft model/Rotational Kinematics/MATLAB Function8 ==
  data: roll input; ZYXquat_inv output; pitch input; yaw input; ZYXquat output
function [ZYXquat_inv,ZYXquat] = Quat_from_Euler(roll,pitch,yaw)
    q_yaw = zeros(4,1);
    q_yaw(1) = cos(yaw/2);
    q_yaw(2:4,1) = sin(yaw/2)*[0 0 1]';

    q_pitch = zeros(4,1);
    q_pitch(1) = cos(pitch/2);
    q_pitch(2:4,1) = sin(pitch/2)*[0 1 0]';

    q_roll = zeros(4,1);
    q_roll(1) = cos(roll/2);
    q_roll(2:4,1) = sin(roll/2)*[1 0 0]';
    
    inv_q_yaw = [q_yaw(1);-q_yaw(2:4)];
    inv_q_pitch = [q_pitch(1);-q_pitch(2:4)];
    inv_q_roll = [q_roll(1);-q_roll(2:4)];

    ZYXquat_inv = quat_mult(quat_mult(inv_q_roll,inv_q_pitch),inv_q_yaw);
    ZYXquat = quat_mult(quat_mult(q_yaw,q_pitch),q_roll);

end

function quat = quat_mult(q1,q2)
    quat = zeros(4,1);
    quat(1) = q1(1)*q2(1)-q1(2)*q2(2)-q1(3)*q2(3)-q1(4)*q2(4);
    quat(2) = q1(1)*q2(2)+q1(2)*q2(1)+q1(3)*q2(4)-q1(4)*q2(3);
    quat(3) = q1(1)*q2(3)-q1(2)*q2(4)+q1(3)*q2(1)+q1(4)*q2(2);
    quat(4) = q1(1)*q2(4)+q1(2)*q2(3)-q1(3)*q2(2)+q1(4)*q2(1);
end

== matlab function ame532Project1_onedrive/9 DoF Dynamic Aircraft model/Rotational Kinematics/MATLAB Function9 ==
  data: q1 input; quat output; q2 input
function quat = quat_mult(q1,q2)
    quat = zeros(4,1);
    quat(1) = q1(1)*q2(1)-q1(2)*q2(2)-q1(3)*q2(3)-q1(4)*q2(4);
    quat(2) = q1(1)*q2(2)+q1(2)*q2(1)+q1(3)*q2(4)-q1(4)*q2(3);
    quat(3) = q1(1)*q2(3)-q1(2)*q2(4)+q1(3)*q2(1)+q1(4)*q2(2);
    quat(4) = q1(1)*q2(4)+q1(2)*q2(3)-q1(3)*q2(2)+q1(4)*q2(1);
end

== matlab function ame532Project1_onedrive/9 DoF Dynamic Aircraft model/Unused tranlational kinmatics/C_EN4 ==
  data: roll input; ZYXDCM output; pitch input; yaw input
function ZYXDCM = DCM_from_Euler(roll,pitch,yaw) % sequence is yaw pitch roll
    yaw_matrix = [cos(yaw) sin(yaw) 0;
                  -sin(yaw) cos(yaw) 0;
                  0 0 1];
    pitch_matrix = [cos(pitch) 0 -sin(pitch);
                    0           1           0;
                    sin(pitch) 0  cos(pitch)];
    roll_matrix = [1            0           0;
                    0          cos(roll)    sin(roll);
                    0           -sin(roll)  cos(roll)];
    ZYXDCM = roll_matrix*pitch_matrix*yaw_matrix;
end

== matlab function ame532Project1_onedrive/9 DoF Dynamic Aircraft model/translational dynamics/MATLAB Function10 ==
  data: p input; Cross_Product_Matrix output; q input; r input
function Cross_Product_Matrix = omega_to_cross_product_matrix(p,q,r)

    Cross_Product_Matrix =[0 -r q; r 0 -p; -q p 0];

end

== matlab function ame532Project1_onedrive/9 DoF Dynamic Aircraft model/aeroforce coefficient block/MATLAB Function ==
  data: AR_matrix input; CL_a output
function CL_a = Calculate_CL_a(AR_matrix)

CL_a = zeros(4,1);

for i = 1:4
    CL_a(i) = 2*pi*(AR_matrix(i)/(2+AR_matrix(i)));
end

== matlab function ame532Project1_onedrive/9 DoF Dynamic Aircraft model/aeroforce coefficient block/extract matrix function2 ==
  data: aero_surface_matrix input; Area_matrix output
function Area_matrix = Extract_Area(aero_surface_matrix)

Area_matrix = aero_surface_matrix(:,6);
end

== matlab function ame532Project1_onedrive/9 DoF Dynamic Aircraft model/Translational Kinematics/new C_EN base on cart. coordinate1 ==
  data: lat input; ZYXDCM output; long input
function ZYXDCM = DCM_from_Euler(lat,long) % sequence of rotation is lat long
%     yaw_matrix = [cos(yaw) sin(yaw) 0;
%                   -sin(yaw) cos(yaw) 0;
%                   0 0 1];
    lat_matrix = [cos(lat) 0 -sin(lat);
                    0           1           0;
                    sin(lat) 0  cos(lat)];
    long_matrix = [1            0           0;
                    0          cos(-long)    sin(-long);
                    0           -sin(-long)  cos(-long)];

    adjust_matrix = [cos(pi/2) 0 -sin(pi/2);
                    0           1           0;
                    sin(pi/2) 0  cos(pi/2)];
    ZYXDCM = adjust_matrix*long_matrix*lat_matrix;
end

%this rotational matrix turns lat long coordinate into a new C_EN
%assuming the N CS is lat and longitudinally rotated, then you would do
%-longditudinal rotation then lat rotation, then rotate 90 degrees again to
%match ECEF

== matlab function ame532Project1_onedrive/9 DoF Dynamic Aircraft model/measurement subsystem/MATLAB Function ==
  data: velocity input; magnitude output
function magnitude = magnitude_from_vector(velocity)

magnitude = sqrt(velocity(1)^2+velocity(2)^2+velocity(3)^2);

end

== matlab function ame532Project1_onedrive/9 DoF Dynamic Aircraft model/mass & aero property calculation/CG calculation ==
  data: M_matrix input; cg_x output; cg_y output; cg_z output
function [cg_x, cg_y, cg_z] = CG_calc(M_matrix)

mass_col = M_matrix(:,1);
x_col = M_matrix(:,5);
y_col = M_matrix(:,6);
z_col = M_matrix(:,7);

cg_x = sum(mass_col.*x_col)/(sum(mass_col));
cg_y = sum(mass_col.*y_col)/(sum(mass_col));
cg_z = sum(mass_col.*z_col)/(sum(mass_col));

end

== matlab function ame532Project1_onedrive/9 DoF Dynamic Aircraft model/mass & aero property calculation/MATLAB Function ==
  data: cg_location input; M_matrix input; J_matrix output
function J_matrix = fcn(cg_location,M_matrix)


mass_col = M_matrix(:,1);
x_dim = M_matrix(:,2);
y_dim = M_matrix(:,3);
z_dim = M_matrix(:,4);
x_loc = M_matrix(:,5);
y_loc = M_matrix(:,6);
z_loc = M_matrix(:,7);

Ixx = zeros(11,1);
Iyy = zeros(11,1);
Izz = zeros(11,1);
Ixz = zeros(11,1);
Izx = Ixz;
Ixy = zeros(11,1);
Iyx = Ixy;
Iyz = zeros(11,1);
Izy = Iyz;

J_matrix = zeros(3,3);

% all moment of inertial is calculated wrt to CG

for i = 1:11
    Ixx(i) = mass_col(i)*(y_dim(i)^2+z_dim(i)^2)/(12)+mass_col(i)*((y_loc(i)-cg_location(2))^2+(z_loc(i)-cg_location(3))^2); % check discussion post
    Iyy(i) = mass_col(i)*(x_dim(i)^2+z_dim(i)^2)/(12)+mass_col(i)*((x_loc(i)-cg_location(1))^2+(z_loc(i)-cg_location(3))^2);
    Izz(i) = mass_col(i)*(y_dim(i)^2+x_dim(i)^2)/(12)+mass_col(i)*((y_loc(i)-cg_location(2))^2+(x_loc(i)-cg_location(1))^2);
    Ixz(i) = mass_col(i)*((z_loc(i)-cg_location(3))*(x_loc(i)-cg_location(1)));
    Ixy(i) = mass_col(i)*((x_loc(i)-cg_location(1))*(y_loc(i)-cg_location(2)));
    Iyz(i) = mass_col(i)*((y_loc(i)-cg_location(2))*(z_loc(i)-cg_location(3)));


end

J_matrix(1,1) = sum(Ixx);
J_matrix(2,2) = sum(Iyy);
J_matrix(3,3) = sum(Izz);
J_matrix(1,2) = sum(Ixy);
J_matrix(2,1) = sum(Ixy);
J_matrix(1,3) = sum(Ixz);
J_matrix(3,1) = sum(Ixz);
J_matrix(2,3) = sum(Iyz);
J_matrix(3,2) = sum(Iyz);

J_matrix = J_matrix./1000;
end

== matlab function ame532Project1_onedrive/9 DoF Dynamic Aircraft model/mass & aero property calculation/MATLAB Function2 ==
  data: M_matrix input; aero_prop output
function aero_prop = fcn(M_matrix)

aero_prop = zeros(4,7);
for i = 1:4
    aero_prop(i,1:3) = M_matrix(i,5:7);
    aero_prop(i,4) = M_matrix(i,2);
end

%% define span for each surface

    aero_prop(1,5) = M_matrix(1,3); %right wing
    aero_prop(2,5) = M_matrix(2,3); %left wing
    aero_prop(3,5) = M_matrix(3,3); %hor stab.
    aero_prop(4,5) = M_matrix(4,4); %ver stab.
%% define area and aspect ratio for each surface

for i = 1:4
    aero_prop(i,6) = aero_prop(i,4)*aero_prop(i,5);
    aero_prop(i,7) = aero_prop(i,5)/aero_prop(i,4);
end

== matlab function ame532Project1_onedrive/9 DoF Dynamic Aircraft model/aeroforce coefficient block/extract matrix function ==
  data: aero_surface_matrix input; AR_matrix output
function AR_matrix = Extract_AR(aero_surface_matrix)

AR_matrix = aero_surface_matrix(:,7);
end

== matlab function ame532Project1_onedrive/9 DoF Dynamic Aircraft model/aeroforce coefficient block/calculatie alpha ==
  data: i0 input; alpha output; v_B input; n_vector input; wind_w input; v_B_BA output; C_BN input
function [alpha,v_B_BA] = fcn(i0,v_B,n_vector,wind_w,C_BN)

alpha = zeros(4,1);
% this function calculates alpha that the aero surface sees

v_B_BA = v_B - C_BN*wind_w;

for i = 1:4
    alpha(i) = i0(i) - asin(dot(v_B_BA,n_vector(:,i))/norm(v_B_BA));
end

== matlab function ame532Project1_onedrive/9 DoF Dynamic Aircraft model/aeroforce coefficient block/MATLAB Function1 ==
  data: CL0 input; CL_s output; CL_a input; alpha input; surface_area input; deflection_angle input
function CL_s = calculate_CL_s(CL0,CL_a,alpha,surface_area,deflection_angle)

CL_s = zeros(4,1);

for i = 1:4
    CL_s(i) = CL0(i)+CL_a(i)*alpha(i)+3*deflection_angle(i)*(0.3);
end

== matlab function ame532Project1_onedrive/9 DoF Dynamic Aircraft model/Rotational Kinematics/MATLAB Function2 ==
  data: phi input; H_matrix_inv output; theta input; psi input
function H_matrix_inv = inv_h_matrix_from_euler(phi,theta,psi)

H_matrix_inv = [1, tan(theta)*sin(phi), tan(theta)*cos(phi);
                0,      cos(phi),           -sin(phi);      
                0,     sin(phi)/cos(theta),   cos(phi)/cos(theta)];

end

== matlab function ame532Project1_onedrive/9 DoF Dynamic Aircraft model/aeroforce coefficient block/MATLAB Function2 ==
  data: CD_0 input; CD_a input; CD_s output; alpha_0 input; alpha input; CL_s input; e input; AR input
function CD_s = calculate_CD_s(CD_0,CD_a,alpha_0,alpha,CL_s,e,AR)
CD_s = zeros(4,1);

for i = 1:4
    
    CD_s(i) = CD_0(i) + CD_a(i)*(alpha(i)-alpha_0(i))^2+(CL_s(i)^2)/(pi*e(i)*AR(i));

end

== matlab function ame532Project1_onedrive/9 DoF Dynamic Aircraft model/aeroforce coefficient block/extract matrix function1 ==
  data: aero_surface_matrix input; AR_matrix output
function AR_matrix = Extract_AR(aero_surface_matrix)

AR_matrix = aero_surface_matrix(:,7);
end

== matlab function ame532Project1_onedrive/9 DoF Dynamic Aircraft model/aeroforce coefficient block/MATLAB Function3 ==
  data: alpha input; CM_0 input; CM_s output; CM_a input
function CM_s = calculate_CM_s(alpha,CM_0,CM_a)

CM_s = zeros(4,1);

for i = 1:4
    CM_s(i) = CM_0(i)+CM_a(i)*alpha(i);
end

== matlab function ame532Project1_onedrive/9 DoF Dynamic Aircraft model/aeroforce & moment block/MATLAB Function ==
  data: CL_s input; Lift_s output; totalspeed input; area_s input
function Lift_s = calculate_Lift_s(CL_s,totalspeed,area_s)

Lift_s = zeros(4,1);
rho = 1.225; %kg/m3

for i = 1:4
    Lift_s(i) = CL_s(i)*0.5*rho*(totalspeed^2)*area_s(i);
end

end

== matlab function ame532Project1_onedrive/9 DoF Dynamic Aircraft model/aeroforce & moment block/MATLAB Function1 ==
  data: aerosurface_matrix input; area_col output
function area_col = extract_area_col(aerosurface_matrix)

area_col = aerosurface_matrix(:,6);

end

== matlab function ame532Project1_onedrive/9 DoF Dynamic Aircraft model/aeroforce & moment block/MATLAB Function2 ==
  data: CD_s input; Drag_s output; totalspeed input; area_s input
function Drag_s = calculate_Drag_s(CD_s,totalspeed,area_s)

Drag_s = zeros(4,1);
rho = 1.225; %kg/m3

for i = 1:4
    Drag_s(i) = CD_s(i)*0.5*rho*(totalspeed^2)*area_s(i);
end

end

== matlab function ame532Project1_onedrive/9 DoF Dynamic Aircraft model/aeroforce & moment block/MATLAB Function3 ==
  data: CM_s input; Moment_s output; totalspeed input; area_s input; chord_s input
function Moment_s = calculate_Moment_s(CM_s,totalspeed,area_s,chord_s)

Moment_s = zeros(4,1);
rho = 1.225; %kg/m3

for i = 1:4
    Moment_s(i) = CM_s(i)*0.5*rho*(totalspeed^2)*area_s(i)*chord_s(i);
end

end

== matlab function ame532Project1_onedrive/9 DoF Dynamic Aircraft model/aeroforce & moment block/MATLAB Function4 ==
  data: aerosurface_matrix input; chord_col output
function chord_col = extract_chord_col(aerosurface_matrix)

chord_col = aerosurface_matrix(:,4);

end

== matlab function ame532Project1_onedrive/9 DoF Dynamic Aircraft model/aeroforce & moment block/MATLAB Function5 ==
  data: Lift_s input; F_w_s output; n_vector_s input; Drag_s input
function F_w_s = Calculate_F_w(Lift_s,n_vector_s,Drag_s)

F_w_s = zeros(3,4);

for i = 1:4
    F_w_s(:,i) = Lift_s(i).*n_vector_s(:,i) - [Drag_s(i) 0 0]';
end

== matlab function ame532Project1_onedrive/9 DoF Dynamic Aircraft model/aeroforce & moment block/MATLAB Function6 ==
  data: n_vector_s input; M_s input; M_w_s output; F_b_s input; x_b_sb input
function M_w_s = Calculate_M_w(n_vector_s,M_s,F_b_s,x_b_sb)

M_w_s = zeros(3,4);

for i = 1:4
      M_w_s(:,i) = M_s(i)*[0 0 0; 0 0 -1; 0 1 0]*n_vector_s(:,i)+cross(x_b_sb(:,i),F_b_s(:,i));
%     M_w_s(:,i) = M_s(i)*[0 0 0; 0 0 -1; 0 1 0]*n_vector_s(:,i)+cross(F_b_s(:,i),x_b_sb(:,i));

end

== matlab function ame532Project1_onedrive/9 DoF Dynamic Aircraft model/Rotational Kinematics/MATLAB Function3 ==
  data: p input; Cross_Product_Matrix output; q input; r input
function Cross_Product_Matrix = omega_to_cross_product_matrix(p,q,r)

    Cross_Product_Matrix =[0 -r q; r 0 -p; -q p 0];

end

== matlab function ame532Project1_onedrive/9 DoF Dynamic Aircraft model/mass & aero property calculation/MATLAB Function1 ==
  data: aero_prop_matrix input; m_matrix input; x_b_s_ac output; cg_location input
function x_b_s_ac = calculate_x_b_sb(aero_prop_matrix,m_matrix,cg_location)
%this function calculates vector of each component to CM of aircraft

x_b_sb = zeros(3,4);
x_b_s_ac = zeros(3,4);
for i = 1:4
    x_b_s_ac(:,i) = m_matrix(i,5:7)' + [0.25*aero_prop_matrix(i,4) 0 0]';
    x_b_s_ac(:,i) = x_b_s_ac(:,i)- cg_location;

%     x_b_sb(:,i) = m_matrix(i,5:7)' - cg_location;

end

== matlab function ame532Project1_onedrive/9 DoF Dynamic Aircraft model/aeroforce & moment block/MATLAB Function7 ==
  data: forcexyz_w_s_matrix input; force_xyz_w output
function force_xyz_w = sum_all_force_xyz(forcexyz_w_s_matrix)

force_xyz_w = zeros(3,1);

for i = 1:3
    force_xyz_w(i) = sum(forcexyz_w_s_matrix(i,:));
end

== matlab function ame532Project1_onedrive/9 DoF Dynamic Aircraft model/aeroforce & moment block/MATLAB Function8 ==
  data: m_b_s input; moments_lmn_b output
function moments_lmn_b = sum_all_moments_b_s(m_b_s)

moments_lmn_b = zeros(3,1);

for i = 1:3
    moments_lmn_b(i) = sum(m_b_s(i,:));
end

== matlab function ame532Project1_onedrive/9 DoF Dynamic Aircraft model/aeroforce & moment block/MATLAB Function9 ==
  data: DCM_WB output; v_body_ba input; alpha output; beta output; v_inf output
function [DCM_WB,alpha,beta,v_inf]  = construct_DCM_bw(v_body_ba)

alpha = atan2(v_body_ba(3),v_body_ba(1));
beta = asin(v_body_ba(2)/norm(v_body_ba));

DCM_WB = [cos(beta) sin(beta) 0; -sin(beta) cos(beta) 0; 0 0 1]*[cos(alpha) 0 sin(alpha); 0 1 0; -sin(alpha) 0 cos(alpha)];
v_inf = norm(v_body_ba);
end

== matlab function ame532Project1_onedrive/9 DoF Dynamic Aircraft model/Rotational Kinematics/MATLAB Function4 ==
  data: DCM input; roll output; pitch output; yaw output
function [roll, pitch, yaw] = Euler_from_DCM(DCM)
   roll = atan2(DCM(2,3),DCM(3,3));
   pitch = -asin(DCM(1,3));
   yaw = atan2(DCM(1,2),DCM(1,1));
end

== matlab function ame532Project1_onedrive/9 DoF Dynamic Aircraft model/Rotational Kinematics/C_EN1 ==
  data: roll input; ZYXDCM output; pitch input; yaw input
function ZYXDCM = DCM_from_Euler(roll,pitch,yaw) % sequence is yaw pitch roll
    yaw_matrix = [cos(yaw) sin(yaw) 0;
                  -sin(yaw) cos(yaw) 0;
                  0 0 1];
    pitch_matrix = [cos(pitch) 0 -sin(pitch);
                    0           1           0;
                    sin(pitch) 0  cos(pitch)];
    roll_matrix = [1            0           0;
                    0          cos(roll)    sin(roll);
                    0           -sin(roll)  cos(roll)];
    ZYXDCM = roll_matrix*pitch_matrix*yaw_matrix;
end

== matlab function ame532Project1_onedrive/9 DoF Dynamic Aircraft model/Rotational Kinematics/C_EN2 ==
  data: roll input; ZYXDCM output; pitch input; yaw input
function ZYXDCM = DCM_from_Euler(roll,pitch,yaw) % sequence is yaw pitch roll
    yaw_matrix = [cos(yaw) -sin(yaw) 0;
                  sin(yaw) cos(yaw) 0;
                  0 0 1];
    pitch_matrix = [cos(pitch) 0 sin(pitch);
                    0           1           0;
                    -sin(pitch) 0  cos(pitch)];
    roll_matrix = [1            0           0;
                    0          cos(roll)    -sin(roll);
                    0           sin(roll)  cos(roll)];
    ZYXDCM = roll_matrix*pitch_matrix*yaw_matrix;
end

== matlab function ame532Project1_onedrive/9 DoF Dynamic Aircraft model/Rotational Kinematics/MATLAB Function5 ==
  data: DCM input; roll output; pitch output; yaw output
function [roll, pitch, yaw] = Euler_from_DCM(DCM)
   roll = atan2(DCM(2,3),DCM(3,3));
   pitch = asin(DCM(1,3));
   yaw = atan2(DCM(1,2),DCM(1,1));
end

== matlab function ame532Project1_onedrive/9 DoF Dynamic Aircraft model/Rotational Kinematics/MATLAB Function6 ==
  data: DCM input; roll output; pitch output; yaw output
function [roll, pitch, yaw] = Euler_from_DCM(DCM)
   roll = atan2(DCM(2,3),DCM(3,3));
   pitch = -asin(DCM(1,3));
   yaw = atan2(DCM(1,2),DCM(1,1));
end

== matlab function ame532Project1_onedrive/9 DoF Dynamic Aircraft model/Rotational Kinematics/MATLAB Function7 ==
  data: quat input; roll output; pitch output; yaw output
function [roll, pitch, yaw] = Euler_from_Quat(quat)
    DCM = zeros(3,3);
    DCM(1) = (quat(1)^2+quat(2)^2-quat(3)^2-quat(4)^2);
    DCM(2) = 2*(quat(2)*quat(3)-quat(1)*quat(4));
    DCM(3) = 2*(quat(2)*quat(4)+quat(1)*quat(3));
    DCM(4) = 2*(quat(2)*quat(3)+quat(1)*quat(4));
    DCM(5) = (quat(1)^2-quat(2)^2+quat(3)^2-quat(4)^2);
    DCM(6) = 2*(quat(3)*quat(4)-quat(1)*quat(2));
    DCM(7) = 2*(quat(2)*quat(4)-quat(1)*quat(3));
    DCM(8) = 2*(quat(3)*quat(4)+quat(1)*quat(2));
    DCM(9) = (quat(1)^2-quat(2)^2-quat(3)^2+quat(4)^2);

    roll = atan2(DCM(2,3),DCM(3,3));
    pitch = -asin(DCM(1,3));
    yaw = atan2(DCM(1,2),DCM(1,1));
end
